simulink model "Multicopter_Testbed"  (R2012b)
settings: Solver=FixedStepDiscrete  SolverMode=SingleTasking  StartTime=0.0  StopTime=inf  FixedStep=Sampletime.Sim  MaxStep=0.005  MinStep=0.0001  RelTol=1e-5
PreLoadFcn:
  | addpath([cd filesep 'Multicopter_Simulation_Data'])
  | initMulticopterSimulationBus;
  | initOveroControlBus;
  | initMulticopterSimulation;
undefined symbols (not defined in the file): Airframe_Pelican, DiscIntNeverNeededParam, Environment_Earth, gcbh, quat_fr_euler, rad, Sampletime, Sensor_Autopilot, vrmfunc
(part 3 of 3)

== system Multicopter_Testbed/Visualisation/VR_View/Quad States to VR_Inputs/Quat to VR ==
  q : Inport
  Mux : Mux  Inputs=2
  NED to VR-vector : Subsystem  mask(Converts NED to VR-vector){}
      mask help: [north east down] => [east up south]
  Quat Decompose : Subsystem  mask(Quaternion Decomposition){}
      mask help:
      | Decomposes a normalized Quaternion into
      | the rotation-vector v and the rotation-angle phi.
  vr_rot : Outport
  wires:
  Mux/1 -> vr_rot/1
  Quat Decompose/1(phi) -> Mux/2
  NED to VR-vector/1(vr) -> Mux/1
  Quat Decompose/2(v) -> NED to VR-vector/1(ned)
  q/1 -> Quat Decompose/1(q)

== system Multicopter_Testbed/Onboard_Control_System/LL_Signal_Processing/IMU_Signal_Processing/LL_Height_Filter/Interval Test ==
  u : Inport
  AND : Logic  AllPortsSameDT=off  OutDataTypeStr=boolean
  FixPt Data Type Duplicate : DataTypeDuplicate  DisableCoverage=on  NumInputPorts=3
  Lower Limit : Constant  DisableCoverage=on  Value=lowlimit  OutDataTypeStr=Inherit: Inherit via back propagation
  Lower Test : RelationalOperator  DisableCoverage=on  Operator=<=  OutDataTypeStr=boolean  ZeroCross=off
  Upper Limit : Constant  DisableCoverage=on  Value=uplimit  OutDataTypeStr=Inherit: Inherit via back propagation
  Upper Test : RelationalOperator  DisableCoverage=on  Operator=<=  OutDataTypeStr=boolean  ZeroCross=off
  y : Outport
  wires:
  AND/1 -> y/1
  u/1 -> Upper Test/1, Lower Test/2, FixPt Data Type Duplicate/1
  Upper Test/1 -> AND/2
  Lower Test/1 -> AND/1
  Upper Limit/1 -> FixPt Data Type Duplicate/3, Upper Test/2
  Lower Limit/1 -> FixPt Data Type Duplicate/2, Lower Test/1

== system Multicopter_Testbed/Visualisation/VR_View/Quad States to VR_Inputs/Euler to VR/Euler to Quat ==
  euler : Inport
  Add : Sum
  Add1 : Sum  Inputs=+-
  Add2 : Sum
  Add3 : Sum  Inputs=+-
  Demux : Demux  Outputs=3
  Gain : Gain  Gain=0.5
  Matrix Concatenate : Concatenate  NumInputs=4  ConcatenateDimension=2
  Product{,1..7} (8 alike) : Product  Inputs=3  RndMeth=Zero
  Trigonometric Function : Trigonometry
  Trigonometric Function1 : Trigonometry  Operator=cos
  Trigonometric Function2 : Trigonometry
  Trigonometric Function3 : Trigonometry  Operator=cos
  Trigonometric Function4 : Trigonometry
  Trigonometric Function5 : Trigonometry  Operator=cos
  q : Outport
  wires:
  euler/1 -> Gain/1
  Gain/1 -> Demux/1
  Demux/3 -> Trigonometric Function4/1, Trigonometric Function5/1  "psi"
  Demux/2 -> Trigonometric Function2/1, Trigonometric Function3/1  "theta"
  Demux/1 -> Trigonometric Function/1, Trigonometric Function1/1  "phi"
  Product/1 -> Add/1
  Product1/1 -> Add/2
  Product2/1 -> Add1/1
  Product3/1 -> Add1/2
  Product4/1 -> Add2/1
  Product5/1 -> Add2/2
  Product6/1 -> Add3/1
  Product7/1 -> Add3/2
  Add/1 -> Matrix Concatenate/1
  Add1/1 -> Matrix Concatenate/2
  Add2/1 -> Matrix Concatenate/3
  Add3/1 -> Matrix Concatenate/4
  Matrix Concatenate/1 -> q/1
  Trigonometric Function5/1 -> Product7/3, Product4/3, Product2/3, Product/3  "c_ps"
  Trigonometric Function2/1 -> Product7/2, Product4/2, Product3/2, Product1/2  "s_th"
  Trigonometric Function/1 -> Product7/1, Product5/1, Product2/1, Product1/1  "s_ph"
  Trigonometric Function4/1 -> Product6/3, Product5/3, Product3/3, Product1/3  "s_ps"
  Trigonometric Function3/1 -> Product6/2, Product5/2, Product2/2, Product/2  "c_th"
  Trigonometric Function1/1 -> Product6/1, Product4/1, Product3/1, Product/1  "c_ph"

== system Multicopter_Testbed/Visualisation/VR_View/Quad States to VR_Inputs/Euler to VR/Quat to VR ==
  q : Inport
  Mux : Mux  Inputs=2
  NED to VR-vector : Subsystem  mask(Converts NED to VR-vector){}
      mask help: [north east down] => [east up south]
  Quat Decompose : Subsystem  mask(Quaternion Decomposition){}
      mask help:
      | Decomposes a normalized Quaternion into
      | the rotation-vector v and the rotation-angle phi.
  vr_rot : Outport
  wires:
  Mux/1 -> vr_rot/1
  Quat Decompose/1(phi) -> Mux/2
  NED to VR-vector/1(vr) -> Mux/1
  Quat Decompose/2(v) -> NED to VR-vector/1(ned)
  q/1 -> Quat Decompose/1(q)

== system Multicopter_Testbed/Visualisation/VR_View/Quad States to VR_Inputs/Quat to VR/NED to VR-vector ==
  ned : Inport
  Gain K*u : Gain  Gain=[0 1 0; 0 0 -1; -1 0 0]  Multiplication=Matrix(K*u)
  vr : Outport
  wires:
  ned/1 -> Gain K*u/1
  Gain K*u/1 -> vr/1

== system Multicopter_Testbed/Visualisation/VR_View/Quad States to VR_Inputs/Quat to VR/Quat Decompose ==
  q : Inport
  Compare To Constant : Subsystem  mask(Compare To Constant){relop=~=, const=1, OutDataTypeStr=uint8, ZeroCross=off}
      mask prompts: relop "Simulink:masks:Operator_MP"; const "Simulink:masks:ConstantValue_MP"; OutDataTypeStr "Simulink:masks:OutputDataType_MP"; ZeroCross "Simulink:masks:EnableZerocrossingDetection_MP"
      mask help: Simulink:masks:CompareToConstant_MD
      mask init: same as Multicopter_Testbed/Ground_Control/Extended_Debug_Demux/Compare To Constant
      mask TypeOptions relop: == | ~= | < | <= | >= | >
      mask TypeOptions OutDataTypeStr: Simulink:masks:uint8 | Simulink:masks:boolean
      mask Callback ZeroCross: sl('zeroCrossEnable', gcbh);
      mask Display: disp(str)
  Constant : Constant  Value=pi  OutDataTypeStr=Inherit: Inherit via back propagation
  Constant1 : Constant  Value=0  VectorParams1D=off
  Constant2 : Constant  Value=[1; 0; 0]  VectorParams1D=off
  Divide : Product  Inputs=*/
  Gain : Gain  Gain=2
  Quat Abs : Subsystem  mask(Absolute value){}
      mask help: sqrt(q(1)^2+q(2)^2+q(3)^2+q(4)^2)
      mask init:
      | pos = get_param(gcb, 'Position');
      | width = pos(3) - pos(1); height = pos(4) - pos(2);
      | fontsize = get_param(gcb, 'fontsize');
      | if fontsize==-1, scale=1; else scale=fontsize/10; end
      mask Display: text(width/2-scale*8, (height/2-scale), '||q||')
  Quat Normalize : Subsystem  mask(Quaternion Normalize){}
      mask help:
      | if abs(q) ~= 0
      |     q_norm = q/sqrt(q(1)^2+q(2)^2+q(3)^2+q(4)^2)
      | else
      |     q_norm = [1; 0; 0; 0]
      |
      | Regrettably implemented in Simulink
      mask init:
      | pos = get_param(gcb, 'Position');
      | width = pos(3) - pos(1); height = pos(4) - pos(2);
      | fontsize = get_param(gcb, 'fontsize');
      | if fontsize==-1, scale=1; else scale=fontsize/10; end
      mask Display:
      | text(width/2-scale*3, (height/2+scale*10), 'q')
      | text(width/2-scale*8, (height/2-scale*6), '||q||')
      | plot([width/2-scale*10 width/2+scale*10], height/2*[1 1])
  Remainder : Math  Operator=mod  SaturateOnIntegerOverflow=on
  Selector : Selector  InputPortWidth=4  IndexOptions=Index vector (dialog)  Indices=[1]  OutputSizes=1
  Selector1 : Selector  InputPortWidth=4  IndexOptions=Index vector (dialog)  Indices=[2 3 4]  OutputSizes=1
  Switch{,1..3} (4 alike) : Switch  Criteria=u2 ~= 0
  Trigonometric Function : Trigonometry  Operator=acos
  Trigonometric Function1 : Trigonometry
  phi : Outport
  v : Outport  Port=2
  wires:
  Divide/1 -> Switch3/1
  Selector1/1 -> Switch3/3, Divide/1
  Switch3/1 -> Switch2/1
  Trigonometric Function1/1 -> Divide/2, Switch3/2
  Constant2/1 -> Switch2/3
  Constant1/1 -> Switch1/3
  Switch2/1 -> v/1
  Switch1/1 -> phi/1
  Gain/1 -> Switch1/1
  Remainder/1 -> Switch2/2, Switch1/2
  Constant/1 -> Remainder/2
  Trigonometric Function/1 -> Trigonometric Function1/1, Gain/1, Remainder/1  "phi_half"
  Selector/1 -> Trigonometric Function/1
  Switch/1 -> Selector1/1, Selector/1
  Quat Normalize/1(q_norm) -> Switch/1
  Compare To Constant/1(y) -> Switch/2
  Quat Abs/1(abs) -> Compare To Constant/1(u)
  q/1 -> Quat Normalize/1(q), Quat Abs/1(q), Switch/3

== system Multicopter_Testbed/Visualisation/VR_View/Quad States to VR_Inputs/Euler to VR/Quat to VR/NED to VR-vector ==
  ned : Inport
  Gain K*u : Gain  Gain=[0 1 0; 0 0 -1; -1 0 0]  Multiplication=Matrix(K*u)
  vr : Outport
  wires:
  ned/1 -> Gain K*u/1
  Gain K*u/1 -> vr/1

== system Multicopter_Testbed/Visualisation/VR_View/Quad States to VR_Inputs/Euler to VR/Quat to VR/Quat Decompose ==
  q : Inport
  Compare To Constant : Subsystem  mask(Compare To Constant){relop=~=, const=1, OutDataTypeStr=uint8, ZeroCross=off}
      mask prompts: relop "Simulink:masks:Operator_MP"; const "Simulink:masks:ConstantValue_MP"; OutDataTypeStr "Simulink:masks:OutputDataType_MP"; ZeroCross "Simulink:masks:EnableZerocrossingDetection_MP"
      mask help: Simulink:masks:CompareToConstant_MD
      mask init: same as Multicopter_Testbed/Ground_Control/Extended_Debug_Demux/Compare To Constant
      mask TypeOptions relop: == | ~= | < | <= | >= | >
      mask TypeOptions OutDataTypeStr: Simulink:masks:uint8 | Simulink:masks:boolean
      mask Callback ZeroCross: sl('zeroCrossEnable', gcbh);
      mask Display: disp(str)
  Constant : Constant  Value=pi  OutDataTypeStr=Inherit: Inherit via back propagation
  Constant1 : Constant  Value=0  VectorParams1D=off
  Constant2 : Constant  Value=[1; 0; 0]  VectorParams1D=off
  Divide : Product  Inputs=*/
  Gain : Gain  Gain=2
  Quat Abs : Subsystem  mask(Absolute value){}
      mask help: sqrt(q(1)^2+q(2)^2+q(3)^2+q(4)^2)
      mask init:
      | pos = get_param(gcb, 'Position');
      | width = pos(3) - pos(1); height = pos(4) - pos(2);
      | fontsize = get_param(gcb, 'fontsize');
      | if fontsize==-1, scale=1; else scale=fontsize/10; end
      mask Display: text(width/2-scale*8, (height/2-scale), '||q||')
  Quat Normalize : Subsystem  mask(Quaternion Normalize){}
      mask help:
      | if abs(q) ~= 0
      |     q_norm = q/sqrt(q(1)^2+q(2)^2+q(3)^2+q(4)^2)
      | else
      |     q_norm = [1; 0; 0; 0]
      |
      | Regrettably implemented in Simulink
      mask init:
      | pos = get_param(gcb, 'Position');
      | width = pos(3) - pos(1); height = pos(4) - pos(2);
      | fontsize = get_param(gcb, 'fontsize');
      | if fontsize==-1, scale=1; else scale=fontsize/10; end
      mask Display:
      | text(width/2-scale*3, (height/2+scale*10), 'q')
      | text(width/2-scale*8, (height/2-scale*6), '||q||')
      | plot([width/2-scale*10 width/2+scale*10], height/2*[1 1])
  Remainder : Math  Operator=mod  SaturateOnIntegerOverflow=on
  Selector : Selector  InputPortWidth=4  IndexOptions=Index vector (dialog)  Indices=[1]  OutputSizes=1
  Selector1 : Selector  InputPortWidth=4  IndexOptions=Index vector (dialog)  Indices=[2 3 4]  OutputSizes=1
  Switch{,1..3} (4 alike) : Switch  Criteria=u2 ~= 0
  Trigonometric Function : Trigonometry  Operator=acos
  Trigonometric Function1 : Trigonometry
  phi : Outport
  v : Outport  Port=2
  wires:
  Divide/1 -> Switch3/1
  Selector1/1 -> Switch3/3, Divide/1
  Switch3/1 -> Switch2/1
  Trigonometric Function1/1 -> Divide/2, Switch3/2
  Constant2/1 -> Switch2/3
  Constant1/1 -> Switch1/3
  Switch2/1 -> v/1
  Switch1/1 -> phi/1
  Gain/1 -> Switch1/1
  Remainder/1 -> Switch2/2, Switch1/2
  Constant/1 -> Remainder/2
  Trigonometric Function/1 -> Trigonometric Function1/1, Gain/1, Remainder/1  "phi_half"
  Selector/1 -> Trigonometric Function/1
  Switch/1 -> Selector1/1, Selector/1
  Quat Normalize/1(q_norm) -> Switch/1
  Compare To Constant/1(y) -> Switch/2
  Quat Abs/1(abs) -> Compare To Constant/1(u)
  q/1 -> Quat Normalize/1(q), Quat Abs/1(q), Switch/3

== system Multicopter_Testbed/Visualisation/VR_View/Quad States to VR_Inputs/Quat to VR/Quat Decompose/Compare To Constant ==
  u : Inport
  Compare : RelationalOperator  Operator=~=  OutDataTypeStr=fixdt(0, 8)  ZeroCross=off  InputSameDT=on
  Constant : Constant  DisableCoverage=on  Value=const  OutDataTypeStr=Inherit: Inherit via back propagation
  y : Outport
  wires:
  u/1 -> Compare/1
  Constant/1 -> Compare/2
  Compare/1 -> y/1

== system Multicopter_Testbed/Visualisation/VR_View/Quad States to VR_Inputs/Quat to VR/Quat Decompose/Quat Abs ==
  q : Inport
  Euclidean_Norm : Subsystem
      mask help: Euclidean Norm
      mask Help: Euclidean Norm
      mask Display: disp('||.||')
  abs : Outport
  wires:
  Euclidean_Norm/1(||u||) -> abs/1
  q/1 -> Euclidean_Norm/1(u)

== system Multicopter_Testbed/Visualisation/VR_View/Quad States to VR_Inputs/Quat to VR/Quat Decompose/Quat Normalize ==
  q : Inport
  Constant : Constant  Value=[1; 0; 0; 0]  VectorParams1D=off  OutDataTypeStr=Inherit: Inherit via back propagation
  Divide : Product  Inputs=*/  OutMin=-1.5  OutMax=1.5  OutDataTypeStr=Inherit: Same as first input
  Quat Abs : Subsystem  mask(Absolute value){}
      mask help: sqrt(q(1)^2+q(2)^2+q(3)^2+q(4)^2)
      mask init:
      | pos = get_param(gcb, 'Position');
      | width = pos(3) - pos(1); height = pos(4) - pos(2);
      | fontsize = get_param(gcb, 'fontsize');
      | if fontsize==-1, scale=1; else scale=fontsize/10; end
      mask Display: text(width/2-scale*8, (height/2-scale), '||q||')
  Switch : Switch  Criteria=u2 ~= 0
  q_norm : Outport
  wires:
  Switch/1 -> q_norm/1
  q/1 -> Quat Abs/1(q), Divide/1
  Quat Abs/1(abs) -> Switch/2, Divide/2
  Divide/1 -> Switch/1
  Constant/1 -> Switch/3

== system Multicopter_Testbed/Visualisation/VR_View/Quad States to VR_Inputs/Euler to VR/Quat to VR/Quat Decompose/Compare To Constant ==
  u : Inport
  Compare : RelationalOperator  Operator=~=  OutDataTypeStr=fixdt(0, 8)  ZeroCross=off  InputSameDT=on
  Constant : Constant  DisableCoverage=on  Value=const  OutDataTypeStr=Inherit: Inherit via back propagation
  y : Outport
  wires:
  u/1 -> Compare/1
  Constant/1 -> Compare/2
  Compare/1 -> y/1

== system Multicopter_Testbed/Visualisation/VR_View/Quad States to VR_Inputs/Euler to VR/Quat to VR/Quat Decompose/Quat Abs ==
  q : Inport
  Euclidean_Norm : Subsystem
      mask help: Euclidean Norm
      mask Help: Euclidean Norm
      mask Display: disp('||.||')
  abs : Outport
  wires:
  Euclidean_Norm/1(||u||) -> abs/1
  q/1 -> Euclidean_Norm/1(u)

== system Multicopter_Testbed/Visualisation/VR_View/Quad States to VR_Inputs/Euler to VR/Quat to VR/Quat Decompose/Quat Normalize ==
  q : Inport
  Constant : Constant  Value=[1; 0; 0; 0]  VectorParams1D=off  OutDataTypeStr=Inherit: Inherit via back propagation
  Divide : Product  Inputs=*/  OutMin=-1.5  OutMax=1.5  OutDataTypeStr=Inherit: Same as first input
  Quat Abs : Subsystem  mask(Absolute value){}
      mask help: sqrt(q(1)^2+q(2)^2+q(3)^2+q(4)^2)
      mask init:
      | pos = get_param(gcb, 'Position');
      | width = pos(3) - pos(1); height = pos(4) - pos(2);
      | fontsize = get_param(gcb, 'fontsize');
      | if fontsize==-1, scale=1; else scale=fontsize/10; end
      mask Display: text(width/2-scale*8, (height/2-scale), '||q||')
  Switch : Switch  Criteria=u2 ~= 0
  q_norm : Outport
  wires:
  Switch/1 -> q_norm/1
  q/1 -> Quat Abs/1(q), Divide/1
  Quat Abs/1(abs) -> Switch/2, Divide/2
  Divide/1 -> Switch/1
  Constant/1 -> Switch/3

== system Multicopter_Testbed/Visualisation/VR_View/Quad States to VR_Inputs/Quat to VR/Quat Decompose/Quat Abs/Euclidean_Norm ==
  u : Inport
  Math Function : Math  Operator=square  SaturateOnIntegerOverflow=on
  Sqrt : Sqrt  SaturateOnIntegerOverflow=on
  Sum of Elements : Sum  Inputs=+
  ||u|| : Outport
  wires:
  u/1 -> Math Function/1
  Math Function/1 -> Sum of Elements/1
  Sum of Elements/1 -> Sqrt/1
  Sqrt/1 -> ||u||/1

== system Multicopter_Testbed/Visualisation/VR_View/Quad States to VR_Inputs/Quat to VR/Quat Decompose/Quat Normalize/Quat Abs ==
  q : Inport
  Euclidean_Norm : Subsystem
      mask help: Euclidean Norm
      mask Help: Euclidean Norm
      mask Display: disp('||.||')
  abs : Outport
  wires:
  Euclidean_Norm/1(||u||) -> abs/1
  q/1 -> Euclidean_Norm/1(u)

== system Multicopter_Testbed/Visualisation/VR_View/Quad States to VR_Inputs/Euler to VR/Quat to VR/Quat Decompose/Quat Abs/Euclidean_Norm ==
  u : Inport
  Math Function : Math  Operator=square  SaturateOnIntegerOverflow=on
  Sqrt : Sqrt  SaturateOnIntegerOverflow=on
  Sum of Elements : Sum  Inputs=+
  ||u|| : Outport
  wires:
  u/1 -> Math Function/1
  Math Function/1 -> Sum of Elements/1
  Sum of Elements/1 -> Sqrt/1
  Sqrt/1 -> ||u||/1

== system Multicopter_Testbed/Visualisation/VR_View/Quad States to VR_Inputs/Euler to VR/Quat to VR/Quat Decompose/Quat Normalize/Quat Abs ==
  q : Inport
  Euclidean_Norm : Subsystem
      mask help: Euclidean Norm
      mask Help: Euclidean Norm
      mask Display: disp('||.||')
  abs : Outport
  wires:
  Euclidean_Norm/1(||u||) -> abs/1
  q/1 -> Euclidean_Norm/1(u)

== system Multicopter_Testbed/Visualisation/VR_View/Quad States to VR_Inputs/Quat to VR/Quat Decompose/Quat Normalize/Quat Abs/Euclidean_Norm ==
  u : Inport
  Math Function : Math  Operator=square  SaturateOnIntegerOverflow=on
  Sqrt : Sqrt  SaturateOnIntegerOverflow=on
  Sum of Elements : Sum  Inputs=+
  ||u|| : Outport
  wires:
  u/1 -> Math Function/1
  Math Function/1 -> Sum of Elements/1
  Sum of Elements/1 -> Sqrt/1
  Sqrt/1 -> ||u||/1

== system Multicopter_Testbed/Visualisation/VR_View/Quad States to VR_Inputs/Euler to VR/Quat to VR/Quat Decompose/Quat Normalize/Quat Abs/Euclidean_Norm ==
  u : Inport
  Math Function : Math  Operator=square  SaturateOnIntegerOverflow=on
  Sqrt : Sqrt  SaturateOnIntegerOverflow=on
  Sum of Elements : Sum  Inputs=+
  ||u|| : Outport
  wires:
  u/1 -> Math Function/1
  Math Function/1 -> Sum of Elements/1
  Sum of Elements/1 -> Sqrt/1
  Sqrt/1 -> ||u||/1
